simulink model "theta_d_meas_circuit"  (R2024b)
settings: Solver=VariableStepAuto  StartTime=0.0  StopTime=10.0  RelTol=1e-3
undefined symbols (not defined in the file): daq, Ts
settings Model: Creator=Enrico  LastModifiedBy=Enrico

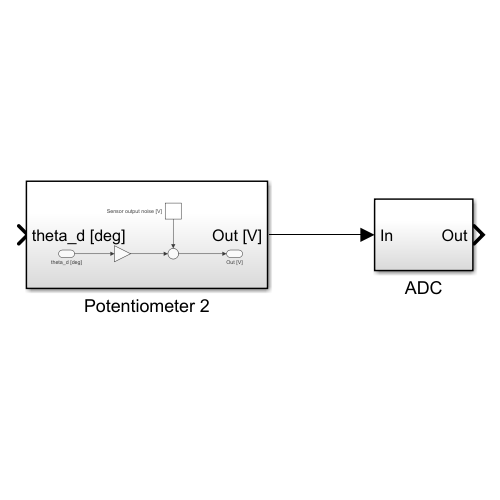
[thumbnail: Simulink's stored preview of the top-level diagram]
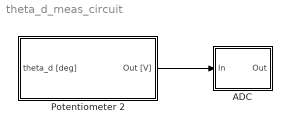
== system theta_d_meas_circuit ==
  ADC : Subsystem
  Potentiometer 2 : Subsystem
  wires:
  Potentiometer 2/1(Out [V]) -> ADC/1(In)

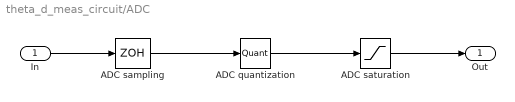
== system theta_d_meas_circuit/ADC ==
  In : Inport
  ADC quantization : Quantizer  QuantizationInterval=daq.adc.q
  ADC sampling : ZeroOrderHold  SampleTime=Ts
  ADC saturation : Saturate  UpperLimit=daq.adc.fs  LowerLimit=-daq.adc.fs
  Out : Outport
  wires:
  ADC quantization/1 -> ADC saturation/1
  In/1 -> ADC sampling/1
  ADC sampling/1 -> ADC quantization/1
  ADC saturation/1 -> Out/1

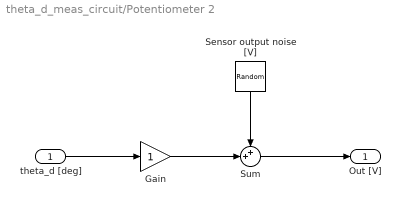
== system theta_d_meas_circuit/Potentiometer 2 ==
  theta_d [deg] : Inport
  Gain : Gain
  Sensor output noise [V] : RandomNumber  SampleTime=Ts
  Sum : Sum  Inputs=++|
  Out [V] : Outport
  wires:
  theta_d [deg]/1 -> Gain/1
  Sum/1 -> Out [V]/1
  Gain/1 -> Sum/2
  Sensor output noise [V]/1 -> Sum/1
